simulink model "AnalisiDinamicastabilitadiunareteelettrica"  (R2024b)
settings: Solver=VariableStepAuto  StartTime=0.0  StopTime=30  RelTol=1e-3
settings Model: NumberOfSteps=2  Creator=jesus  LastModifiedBy=jesus

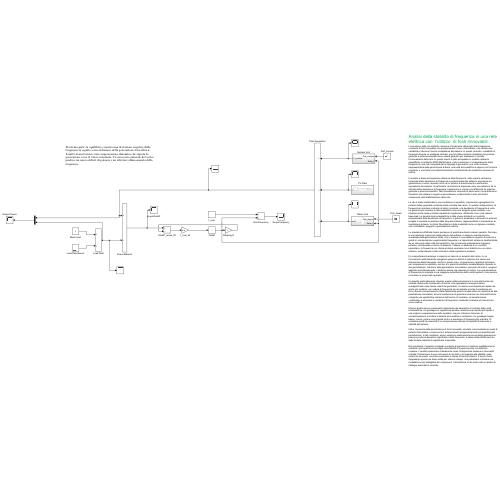
[thumbnail: Simulink's stored preview of the top-level diagram]
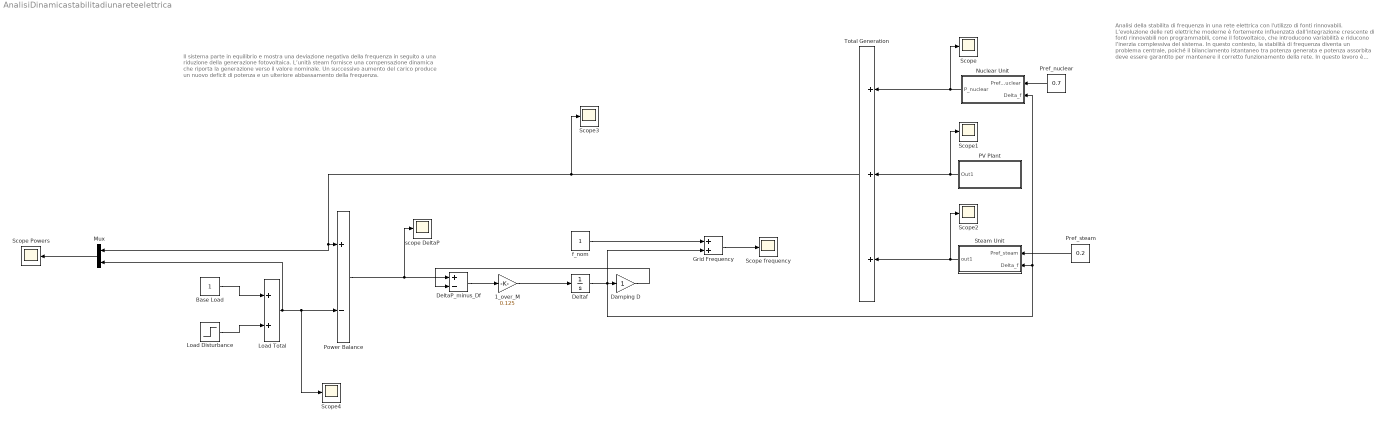
== system AnalisiDinamicastabilitadiunareteelettrica ==
  note: Analisi della stabilita di frequenza in una rete elettrica con l'utilizzo di fonti rinnovabili.
      | L’evoluzione delle reti elettriche moderne è fortemente influenzata dall’integrazione crescente di fonti rinnovabili non programmabili, come il fotovoltaico, che introducono variabilità e riducono l’inerzia complessiva del sistema. In questo contesto, la stabilità di frequenza diventa un problema centrale, poiché il bilanciamento istantaneo tra potenza generata e potenza assorbita deve essere garantito per mantenere il corretto funzionamento della rete. In questo lavoro è stato sviluppato un modello dinamico semplificato in ambiente MATLAB/Simulink, volto a descrivere il comportamento della frequenza in una rete composta da tre tipologie di generatori: una unità nucleare, rappresentativa della generazione di base, una unità termoelettrica a vapore con funzione regolante, e una fonte rinnovabile fotovoltaica caratterizzata da variabilità e assenza di inerzia.
      | Il modello si basa sull’equazione dinamica della frequenza, nella quale la variazione temporale della deviazione di frequenza è proporzionale allo sbilancio di potenza tra generazione e carico, tenendo conto di un termine di smorzamento e dell’inerzia equivalente del sistema. In particolare, la dinamica è espressa come una relazione tra la derivata della deviazione di frequenza, il parametro di inerzia e la differenza tra potenza generata e potenza assorbita. Tale formulazione consente di descrivere il comportamento transitorio del sistema in seguito a perturbazioni, evidenziando il ruolo dei diversi componenti nella stabilizzazione della rete.
      | La rete è stata inizializzata in una condizione di equilibrio, imponendo l’uguaglianza tra potenza totale generata e potenza totale richiesta dal carico. In questa configurazione, la frequenza si mantiene costante al valore nominale, e la deviazione di frequenza è nulla. La generazione nucleare è stata modellata come una sorgente quasi costante, con dinamica molto lenta e limitata capacità di regolazione, riflettendo il suo ruolo reale di base-load. La generazione termoelettrica è stata invece dotata di un controllo proporzionale sulla deviazione di frequenza, in grado di aumentare o diminuire la potenza erogata in risposta a variazioni della frequenza stessa, rappresentando il meccanismo di regolazione primaria. La fonte fotovoltaica è stata modellata come un ingresso variabile, non controllabile, soggetto a perturbazioni esterne.
      | Le simulazioni effettuate hanno permesso di analizzare diversi scenari operativi. Nel caso di una riduzione improvvisa della potenza fotovoltaica, si osserva una diminuzione immediata della generazione totale, che si traduce in uno sbilancio negativo di potenza e quindi in una deviazione negativa della frequenza. La risposta del sistema è caratterizzata da un intervento della unità termoelettrica, che incrementa gradualmente la propria potenza, contribuendo a ridurre lo sbilancio. Tuttavia, in assenza di un controllo secondario, la frequenza non ritorna al valore nominale ma si stabilizza su un valore inferiore, evidenziando il limite intrinseco della regolazione primaria.
      | Un comportamento analogo si osserva nel caso di un aumento del carico, in cui l’incremento della domanda energetica genera un deficit di potenza che causa una diminuzione della frequenza. Anche in questo caso, la generazione regolante interviene per compensare lo squilibrio, ma non è in grado di annullarlo completamente. Quando le due perturbazioni, riduzione della generazione rinnovabile e aumento del carico, vengono applicate simultaneamente, il sistema mostra una risposta più critica, con una deviazione di frequenza più marcata e una maggiore sollecitazione delle unità regolanti, che possono avvicinarsi ai propri limiti operativi.
      | Un aspetto particolarmente rilevante emerso dalle simulazioni è il ruolo dell’inerzia del sistema. Riducendo il parametro di inerzia, che rappresenta l’energia cinetica immagazzinata nelle masse rotanti dei generatori, si osserva una risposta più rapida ma anche più instabile, con cadute di frequenza più accentuate e tempi di variazione più brevi. Questo comportamento riflette fedelmente quanto accade nelle reti moderne ad alta penetrazione rinnovabile, dove la sostituzione di generatori sincroni con fonti elettroniche comporta una significativa riduzione dell’inerzia. Al contrario, un’elevata inerzia contribuisce a smorzare le variazioni di frequenza, rendendo il sistema più robusto ma meno reattivo.
      | Ulteriori analisi hanno evidenziato l’importanza del parametro di controllo della unità termoelettrica. Un guadagno di regolazione elevato consente una risposta più rapida e una migliore compensazione dello squilibrio, ma può introdurre fenomeni di sovraelongazione e rendere il sistema più sensibile a oscillazioni. Un guadagno troppo basso, invece, porta a una risposta lenta e a deviazioni di frequenza più marcate. Si evidenzia quindi la necessità di un compromesso ottimale tra rapidità di intervento e stabilità del sistema.
      | Infine, l’aumento della penetrazione di fonti rinnovabili, simulato incrementando la quota di potenza fotovoltaica, mostra come il sistema diventi progressivamente più sensibile alle perturbazioni. In tali condizioni, anche variazioni relativamente piccole della generazione possono produrre deviazioni significative della frequenza, a causa della ridotta inerzia e della limitata capacità di regolazione immediata.
      | Nel complesso, il modello sviluppato consente di riprodurre in maniera qualitativamente realistica i principali fenomeni legati alla stabilità di frequenza nelle reti elettriche moderne. I risultati evidenziano chiaramente come l’integrazione massiva di rinnovabili richieda l’introduzione di nuovi strumenti di controllo e di supporto alla stabilità, quali sistemi di accumulo, controllo secondario e risorse di inerzia sintetica. Il lavoro svolto rappresenta quindi una base solida per ulteriori sviluppi, che potrebbero includere una modellazione più dettagliata dei componenti, l’introduzione di reti multi-nodo e l’analisi di strategie avanzate di controllo.
  note: Il sistema parte in equilibrio e mostra una deviazione negativa della frequenza in seguito a una riduzione della generazione fotovoltaica. L’unità steam fornisce una compensazione dinamica che riporta la generazione verso il valore nominale. Un successivo aumento del carico produce un nuovo deficit di potenza e un ulteriore abbassamento della frequenza.
  1_over_M : Gain  Gain=0.125
  Base Load : Constant
  Damping D : Gain
  DeltaP_minus_Df : Sum  Inputs=+-
  Deltaf : Integrator
  Grid Frequency : Sum
  Load Disturbance : Step  Time=10  After=0.05  SampleTime=0
  Load Total : Sum
  Mux : Mux  Inputs=2
  Nuclear Unit : Subsystem
  PV Plant : Subsystem
  Power Balance : Sum  Inputs=+-
  Pref_nuclear : Constant  Value=0.7
  Pref_steam : Constant  Value=0.2
  Scope{,1..4} (5 alike) : Scope
  Scope Powers : Scope
  Scope frequency : Scope
  Steam Unit : Subsystem
  Total Generation : Sum  Inputs=+++
  f_nom : Constant
  scope DeltaP : Scope
  wires:
  Load Disturbance/1 -> Load Total/2
  Base Load/1 -> Load Total/1
  Power Balance/1 -> scope DeltaP/1, DeltaP_minus_Df/1
  Deltaf/1 -> Grid Frequency/2, Nuclear Unit/2(Delta_f), Steam Unit/2(Delta_f), Damping D/1
  DeltaP_minus_Df/1 -> 1_over_M/1
  1_over_M/1 -> Deltaf/1
  f_nom/1 -> Grid Frequency/1
  Load Total/1 -> Mux/2, Scope4/1, Power Balance/2
  Grid Frequency/1 -> Scope frequency/1
  Mux/1 -> Scope Powers/1
  Total Generation/1 -> Scope3/1, Mux/1, Power Balance/1
  Nuclear Unit/1(P_nuclear) -> Scope/1, Total Generation/1
  Steam Unit/1(out1) -> Scope2/1, Total Generation/3
  PV Plant/1(Out1) -> Scope1/1, Total Generation/2
  Pref_steam/1 -> Steam Unit/1(Pref_steam)
  Damping D/1 -> DeltaP_minus_Df/2
  Pref_nuclear/1 -> Nuclear Unit/1(Pref_nuclear)

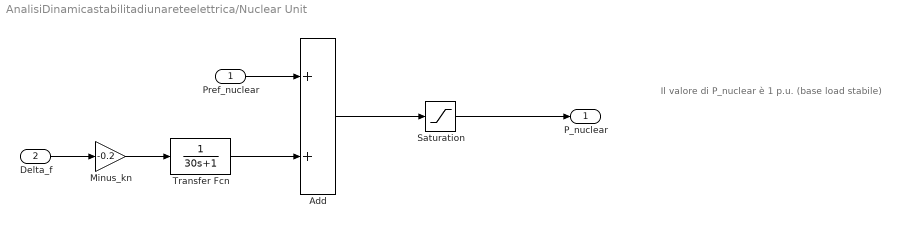
== system AnalisiDinamicastabilitadiunareteelettrica/Nuclear Unit ==
  note: Il valore di P_nuclear è 1 p.u. (base load stabile)
  Pref_nuclear : Inport
  Delta_f : Inport  Port=2
  Add : Sum
  Minus_kn : Gain  Gain=-0.2
  Saturation : Saturate  UpperLimit=0.8  LowerLimit=0.6
  Transfer Fcn : TransferFcn  Denominator=[30 1]
  P_nuclear : Outport
  wires:
  Pref_nuclear/1 -> Add/1
  Delta_f/1 -> Minus_kn/1
  Minus_kn/1 -> Transfer Fcn/1
  Transfer Fcn/1 -> Add/2
  Add/1 -> Saturation/1
  Saturation/1 -> P_nuclear/1

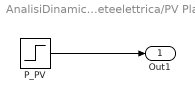
== system AnalisiDinamicastabilitadiunareteelettrica/PV Plant ==
  P_PV : Step  Time=5  Before=0.1  After=0.05  SampleTime=0
  Out1 : Outport
  wires:
  P_PV/1 -> Out1/1

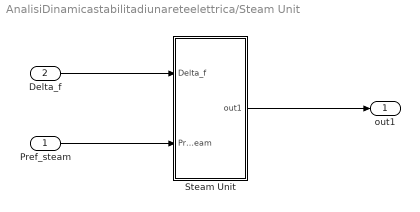
== system AnalisiDinamicastabilitadiunareteelettrica/Steam Unit ==
  Pref_steam : Inport
  Delta_f : Inport  Port=2
  Steam Unit : Subsystem
  out1 : Outport
  wires:
  Steam Unit/1(out1) -> out1/1
  Delta_f/1 -> Steam Unit/1(Delta_f)
  Pref_steam/1 -> Steam Unit/2(Pref_steam)

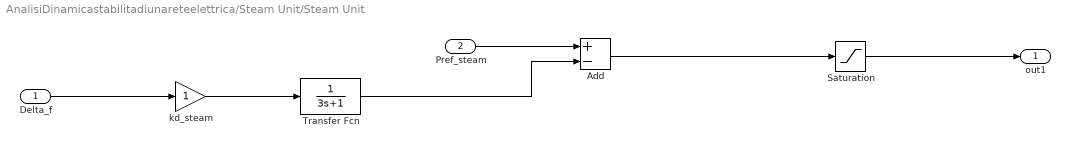
== system AnalisiDinamicastabilitadiunareteelettrica/Steam Unit/Steam Unit ==
  Delta_f : Inport
  Pref_steam : Inport  Port=2
  Add : Sum  Inputs=+-
  Saturation : Saturate  UpperLimit=0.3  LowerLimit=0
  Transfer Fcn : TransferFcn  Denominator=[3 1]
  kd_steam : Gain
  out1 : Outport
  wires:
  Pref_steam/1 -> Add/1
  Delta_f/1 -> kd_steam/1
  Saturation/1 -> out1/1
  kd_steam/1 -> Transfer Fcn/1
  Transfer Fcn/1 -> Add/2
  Add/1 -> Saturation/1
